simulink model "Electrical_System_2018b_obfs"  (R2019b)
settings: Solver=VariableStepAuto  StartTime=0.0  StopTime=5  RelTol=1e-3  AbsTol=1e-3  EnableMultiTasking=on
InitFcn:
  | Steady_State_Initialisation;
StopFcn:
  | %sscexplore(simlog);
  | %Logging
undefined symbols (not defined in the file): abrlhklxvp, aexgmhuedq, afmfmjnutg, afpphrjpnc, ahuxbyvruc, alarvljztt, amxnyqmnuw, aodrlwvqie, aolhmuplyq, aqpmguuqkg, auesgwirzl, aurophlnng, awamelrhru, ayfhvxflxn, azxkacuhqc, babszerikg, bawhdqanwq, bevoqecvei, bltjvqbchx, bmqsuewujl, bsmyqjfgnf, btvjbsmnve, bywgxqeadw, bziaduxaer, bzmcmdqocb, bzsvyvetat, ccsjnrbsih, cdvenygxwh, cedkrnslhx, cjheorclzs, cjrdshrtqx, ckhavyhcza, ckxewznhlz, cmrcgyiplk, conenicnws, cqkejbgjnn, csfnuwymhe, cunupkhwbh, cwzfvzuxxh, dcadmadufn, dcfponivnv, ddtrqjrhjn, dfhoxvkqas, dfrhtcwpne, dfvomcagjv, djijwylxea, dnmeqksrrm, dnzewbdkaa, dsqcykyxav, dtswwlttmm, ecumpidjtv, edegaywrct, ejjjsmnejc, eknqnehjdz, emvdetzouf, esxbqkbahr, etnkkbreiq, eunoiiiirw, ewewcuedir, fatkfxdhtc ... (+386)
libraries: fl_lib x802, ee_lib x362, fl_ps_legacy_lib x160, nesl_utility x85
(part 3 of 26)

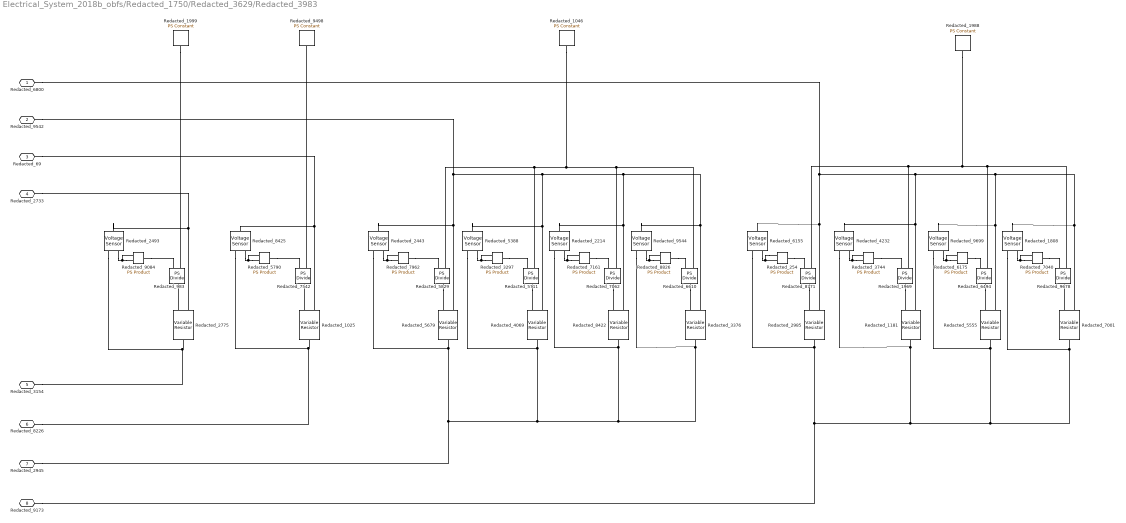
== system Electrical_System_2018b_obfs/Redacted_1750/Redacted_3629/Redacted_3983 ==
  Redacted_1025 : fl_lib/Electrical/Electrical Elements/Variable Resistor  Rmin=qncggggexc Ohm  i_specify=off  i_priority=None  i=gwvltjgfle A  i_nominal_specify=off  i_nominal_unit=A  i_nominal_value=ddwygaqqls  v_specify=off  v_priority=None  v=xwdlpdmsta V  v_nominal_specify=off  v_nominal_unit=V  v_nominal_value=czztgpkpzk
  Redacted_1046 : fl_lib/Physical Signals/Sources/PS Constant  constant=yrrhxgjxjc
  Redacted_1181 : fl_lib/Electrical/Electrical Elements/Variable Resistor  Rmin=nictvldxmh Ohm  i_specify=off  i_priority=None  i=znkaguzczs A  i_nominal_specify=off  i_nominal_unit=A  i_nominal_value=gwvbwqzrqi  v_specify=off  v_priority=None  v=zswwklaalm V  v_nominal_specify=off  v_nominal_unit=V  v_nominal_value=yhsekcleki
  Redacted_{1808,2214,2443,2493,4232,5388,6155,8425,9544,9699} (10 alike) : fl_lib/Electrical/Electrical Sensors/Voltage Sensor
  Redacted_{983,1969,5711,5829,6494,6610,7062,7542,8771,9678} (10 alike) : fl_ps_legacy_lib/Legacy Physical Signals/Functions/PS Divide
      settings: SourceProductName=Simscape  SourceProductBaseCode=SS  InternalSimscapePortConfiguration="{\"Bottom\":[],\"Left\":[{\"id\":\"I1\",\"label\":\"\",\"type\":\"input\"},{\"id\":\"I2\",\"label\":\"\",\"type\":\"input\"}],\"Right\":[{\"id\":\"O\",\"label\":\"\",\"type\":\"output\"}],\"Top\":[]}"
  Redacted_1988 : fl_lib/Physical Signals/Sources/PS Constant  constant=dwzkorkybi
  Redacted_1999 : fl_lib/Physical Signals/Sources/PS Constant  constant=qaltaheucg
  Redacted_{254,3297,3744,5790,6175,7040,7161,7962,8826,9084} (10 alike) : fl_ps_legacy_lib/Legacy Physical Signals/Functions/PS Product
      settings: SourceProductName=Simscape  SourceProductBaseCode=SS
  Redacted_2775 : fl_lib/Electrical/Electrical Elements/Variable Resistor  Rmin=reyjghhurh Ohm  i_specify=off  i_priority=None  i=fnfcgkgufq A  i_nominal_specify=off  i_nominal_unit=A  i_nominal_value=ruiumlemge  v_specify=off  v_priority=None  v=rpfslwjagr V  v_nominal_specify=off  v_nominal_unit=V  v_nominal_value=kprgkhsdzv
  Redacted_2985 : fl_lib/Electrical/Electrical Elements/Variable Resistor  Rmin=opektvarcr Ohm  i_specify=off  i_priority=None  i=ipmwytsvba A  i_nominal_specify=off  i_nominal_unit=A  i_nominal_value=zmaalwbitl  v_specify=off  v_priority=None  v=mourxlmgxq V  v_nominal_specify=off  v_nominal_unit=V  v_nominal_value=olwmmtumto
  Redacted_3376 : fl_lib/Electrical/Electrical Elements/Variable Resistor  Rmin=dmoucclhwu Ohm  i_specify=off  i_priority=None  i=qsvqtyyrfy A  i_nominal_specify=off  i_nominal_unit=A  i_nominal_value=ejaoihdkoa  v_specify=off  v_priority=None  v=bjbzrdorum V  v_nominal_specify=off  v_nominal_unit=V  v_nominal_value=hihsrnonml
  Redacted_4069 : fl_lib/Electrical/Electrical Elements/Variable Resistor  Rmin=bbvrroiejc Ohm  i_specify=off  i_priority=None  i=wnccttposb A  i_nominal_specify=off  i_nominal_unit=A  i_nominal_value=dxfjwicvev  v_specify=off  v_priority=None  v=rbnooizcor V  v_nominal_specify=off  v_nominal_unit=V  v_nominal_value=vmgjehqswm
  Redacted_5555 : fl_lib/Electrical/Electrical Elements/Variable Resistor  Rmin=dsgwiuwtzd Ohm  i_specify=off  i_priority=None  i=qbydpwndjg A  i_nominal_specify=off  i_nominal_unit=A  i_nominal_value=olcbtcjicg  v_specify=off  v_priority=None  v=jvfxdepjcq V  v_nominal_specify=off  v_nominal_unit=V  v_nominal_value=claoggoaet
  Redacted_5679 : fl_lib/Electrical/Electrical Elements/Variable Resistor  Rmin=alpgflrfvh Ohm  i_specify=off  i_priority=None  i=hhwawqdbpi A  i_nominal_specify=off  i_nominal_unit=A  i_nominal_value=hmlbwyynal  v_specify=off  v_priority=None  v=mblpeolwgc V  v_nominal_specify=off  v_nominal_unit=V  v_nominal_value=fswqhenwkq
  Redacted_7001 : fl_lib/Electrical/Electrical Elements/Variable Resistor  Rmin=wojwfybect Ohm  i_specify=off  i_priority=None  i=cubmhvxrnv A  i_nominal_specify=off  i_nominal_unit=A  i_nominal_value=jjakzqrkrp  v_specify=off  v_priority=None  v=kgoihxmpfv V  v_nominal_specify=off  v_nominal_unit=V  v_nominal_value=dzhpomehap
  Redacted_8422 : fl_lib/Electrical/Electrical Elements/Variable Resistor  Rmin=eatydowpoa Ohm  i_specify=off  i_priority=None  i=pfhnarewmr A  i_nominal_specify=off  i_nominal_unit=A  i_nominal_value=mvkwcnovui  v_specify=off  v_priority=None  v=vbpjazytgn V  v_nominal_specify=off  v_nominal_unit=V  v_nominal_value=ttjtmxbkxy
  Redacted_9498 : fl_lib/Physical Signals/Sources/PS Constant  constant=ljceyavbcj
  Redacted_6800 : PMIOPort  Side=Left
  Redacted_9542 : PMIOPort  Port=2  Side=Left
  Redacted_69 : PMIOPort  Port=3  Side=Left
  Redacted_2733 : PMIOPort  Port=4  Side=Left
  Redacted_3154 : PMIOPort  Port=5  Side=Left
  Redacted_8226 : PMIOPort  Port=6  Side=Left
  Redacted_2945 : PMIOPort  Port=7  Side=Left
  Redacted_9173 : PMIOPort  Port=8  Side=Left
  connections:
  Redacted_254/LConn1 -- Redacted_254/LConn2 -- Redacted_6155/RConn1
  Redacted_3744/LConn2 -- Redacted_3744/LConn1 -- Redacted_4232/RConn1
  Redacted_6494/LConn2 -- Redacted_9678/LConn2 -- Redacted_1988/RConn1 -- Redacted_8771/LConn2 -- Redacted_1969/LConn2
  Redacted_5679/RConn1 -- Redacted_2443/RConn2 -- Redacted_2945/RConn1 -- Redacted_9544/RConn2 -- Redacted_3376/RConn1 -- Redacted_2214/RConn2 -- Redacted_8422/RConn1 -- Redacted_4069/RConn1 -- Redacted_5388/RConn2
  Redacted_1025/LConn2 -- Redacted_8425/LConn1 -- Redacted_69/RConn1
  Redacted_1181/LConn2 -- Redacted_4232/LConn1 -- Redacted_6800/RConn1 -- Redacted_6155/LConn1 -- Redacted_2985/LConn2 -- Redacted_1808/LConn1 -- Redacted_7001/LConn2 -- Redacted_5555/LConn2 -- Redacted_9699/LConn1
  Redacted_2493/RConn2 -- Redacted_2775/RConn1 -- Redacted_3154/RConn1
  Redacted_8425/RConn2 -- Redacted_1025/RConn1 -- Redacted_8226/RConn1
  Redacted_8826/LConn2 -- Redacted_8826/LConn1 -- Redacted_9544/RConn1
  Redacted_9699/RConn2 -- Redacted_5555/RConn1 -- Redacted_9173/RConn1 -- Redacted_2985/RConn1 -- Redacted_6155/RConn2 -- Redacted_4232/RConn2 -- Redacted_1181/RConn1 -- Redacted_7001/RConn1 -- Redacted_1808/RConn2
  Redacted_5790/LConn2 -- Redacted_5790/LConn1 -- Redacted_8425/RConn1
  Redacted_7040/LConn2 -- Redacted_7040/LConn1 -- Redacted_1808/RConn1
  Redacted_2214/LConn1 -- Redacted_8422/LConn2 -- Redacted_9544/LConn1 -- Redacted_3376/LConn2 -- Redacted_4069/LConn2 -- Redacted_5388/LConn1 -- Redacted_9542/RConn1 -- Redacted_5679/LConn2 -- Redacted_2443/LConn1
  Redacted_3297/LConn2 -- Redacted_3297/LConn1 -- Redacted_5388/RConn1
  Redacted_7062/LConn2 -- Redacted_6610/LConn2 -- Redacted_1046/RConn1 -- Redacted_5829/LConn2 -- Redacted_5711/LConn2
  Redacted_2493/LConn1 -- Redacted_2775/LConn2 -- Redacted_2733/RConn1
  Redacted_7161/LConn2 -- Redacted_7161/LConn1 -- Redacted_2214/RConn1
  Redacted_9084/LConn2 -- Redacted_9084/LConn1 -- Redacted_2493/RConn1
  Redacted_7962/LConn2 -- Redacted_7962/LConn1 -- Redacted_2443/RConn1
  Redacted_6175/LConn2 -- Redacted_6175/LConn1 -- Redacted_9699/RConn1
  Redacted_3297/RConn1 -- Redacted_5711/LConn1
  Redacted_1025/LConn1 -- Redacted_7542/RConn1
  Redacted_3744/RConn1 -- Redacted_1969/LConn1
  Redacted_6175/RConn1 -- Redacted_6494/LConn1
  Redacted_5829/RConn1 -- Redacted_5679/LConn1
  Redacted_1969/RConn1 -- Redacted_1181/LConn1
  Redacted_9084/RConn1 -- Redacted_983/LConn1
  Redacted_7161/RConn1 -- Redacted_7062/LConn1
  Redacted_8771/RConn1 -- Redacted_2985/LConn1
  Redacted_8826/RConn1 -- Redacted_6610/LConn1
  Redacted_7542/LConn2 -- Redacted_9498/RConn1
  Redacted_254/RConn1 -- Redacted_8771/LConn1
  Redacted_2775/LConn1 -- Redacted_983/RConn1
  Redacted_1999/RConn1 -- Redacted_983/LConn2
  Redacted_7001/LConn1 -- Redacted_9678/RConn1
  Redacted_5711/RConn1 -- Redacted_4069/LConn1
  Redacted_7962/RConn1 -- Redacted_5829/LConn1
  Redacted_6494/RConn1 -- Redacted_5555/LConn1
  Redacted_7062/RConn1 -- Redacted_8422/LConn1
  Redacted_5790/RConn1 -- Redacted_7542/LConn1
  Redacted_6610/RConn1 -- Redacted_3376/LConn1
  Redacted_7040/RConn1 -- Redacted_9678/LConn1

== system Electrical_System_2018b_obfs/Redacted_1750/Redacted_393/Redacted_3640 ==
  Redacted_1716 : fl_lib/Physical Signals/Sources/PS Constant  constant=mmajduezkq
  Redacted_199 : fl_ps_legacy_lib/Legacy Physical Signals/Functions/PS Divide
      settings: SourceProductName=Simscape  SourceProductBaseCode=SS  InternalSimscapePortConfiguration="{\"Bottom\":[],\"Left\":[{\"id\":\"I1\",\"label\":\"\",\"type\":\"input\"},{\"id\":\"I2\",\"label\":\"\",\"type\":\"input\"}],\"Right\":[{\"id\":\"O\",\"label\":\"\",\"type\":\"output\"}],\"Top\":[]}"
  Redacted_4562 : fl_lib/Electrical/Electrical Elements/Variable Resistor  Rmin=kdjcxtkztl Ohm  i_specify=off  i_priority=None  i=cqxgsgfmtn A  i_nominal_specify=off  i_nominal_unit=A  i_nominal_value=bklpitcnvv  v_specify=off  v_priority=None  v=hyuagysdcb V  v_nominal_specify=off  v_nominal_unit=V  v_nominal_value=etqsntubpw
  Redacted_4611 : fl_lib/Electrical/Electrical Elements/Variable Resistor  Rmin=tgyotuwxyj Ohm  i_specify=off  i_priority=None  i=ffbyfrgsin A  i_nominal_specify=off  i_nominal_unit=A  i_nominal_value=lmnpciehqe  v_specify=off  v_priority=None  v=veajvkhyvt V  v_nominal_specify=off  v_nominal_unit=V  v_nominal_value=boksjqkemi
  Redacted_4847 : fl_ps_legacy_lib/Legacy Physical Signals/Functions/PS Product
      settings: SourceProductName=Simscape  SourceProductBaseCode=SS
  Redacted_5241 : fl_lib/Physical Signals/Sources/PS Constant  constant=uldbrsmhhe
  Redacted_5245 : fl_lib/Electrical/Electrical Sensors/Voltage Sensor
  Redacted_6942 : fl_lib/Electrical/Electrical Sensors/Voltage Sensor
  Redacted_8381 : fl_ps_legacy_lib/Legacy Physical Signals/Functions/PS Divide
      settings: SourceProductName=Simscape  SourceProductBaseCode=SS  InternalSimscapePortConfiguration="{\"Bottom\":[],\"Left\":[{\"id\":\"I1\",\"label\":\"\",\"type\":\"input\"},{\"id\":\"I2\",\"label\":\"\",\"type\":\"input\"}],\"Right\":[{\"id\":\"O\",\"label\":\"\",\"type\":\"output\"}],\"Top\":[]}"
  Redacted_9241 : fl_ps_legacy_lib/Legacy Physical Signals/Functions/PS Product
      settings: SourceProductName=Simscape  SourceProductBaseCode=SS
  Redacted_8912 : PMIOPort  Side=Left
  Redacted_9942 : PMIOPort  Port=2  Side=Left
  Redacted_6824 : PMIOPort  Port=3  Side=Left
  Redacted_5238 : PMIOPort  Port=4  Side=Left
  connections:
  Redacted_9241/LConn1 -- Redacted_9241/LConn2 -- Redacted_6942/RConn1
  Redacted_6942/LConn1 -- Redacted_4562/LConn2 -- Redacted_8912/RConn1
  Redacted_5245/RConn2 -- Redacted_4611/RConn1 -- Redacted_6824/RConn1
  Redacted_4847/LConn1 -- Redacted_5245/RConn1 -- Redacted_4847/LConn2
  Redacted_4562/RConn1 -- Redacted_6942/RConn2 -- Redacted_5238/RConn1
  Redacted_5245/LConn1 -- Redacted_4611/LConn2 -- Redacted_9942/RConn1
  Redacted_8381/LConn2 -- Redacted_5241/RConn1
  Redacted_199/RConn1 -- Redacted_4562/LConn1
  Redacted_9241/RConn1 -- Redacted_199/LConn1
  Redacted_4847/RConn1 -- Redacted_8381/LConn1
  Redacted_1716/RConn1 -- Redacted_199/LConn2
  Redacted_8381/RConn1 -- Redacted_4611/LConn1

== system Electrical_System_2018b_obfs/Redacted_1750/Redacted_418/Redacted_6987 ==
  Redacted_2047 : fl_lib/Electrical/Electrical Elements/Variable Resistor  Rmin=lauxoojxid Ohm  i_specify=off  i_priority=None  i=plucywvrmo A  i_nominal_specify=off  i_nominal_unit=A  i_nominal_value=pntbnmmjvt  v_specify=off  v_priority=None  v=exyxduxjmg V  v_nominal_specify=off  v_nominal_unit=V  v_nominal_value=uxkjompdua
  Redacted_2337 : fl_lib/Electrical/Electrical Sensors/Voltage Sensor
  Redacted_2505 : fl_lib/Electrical/Electrical Elements/Variable Resistor  Rmin=vmtqcufeiw Ohm  i_specify=off  i_priority=None  i=jdptkrmseg A  i_nominal_specify=off  i_nominal_unit=A  i_nominal_value=gpzxlmwhqh  v_specify=off  v_priority=None  v=yfdhwgbouy V  v_nominal_specify=off  v_nominal_unit=V  v_nominal_value=fbrxqazbqz
  Redacted_2649 : fl_lib/Physical Signals/Sources/PS Constant  constant=oimdssqwfz
  Redacted_3101 : fl_ps_legacy_lib/Legacy Physical Signals/Functions/PS Divide
      settings: SourceProductName=Simscape  SourceProductBaseCode=SS  InternalSimscapePortConfiguration="{\"Bottom\":[],\"Left\":[{\"id\":\"I1\",\"label\":\"\",\"type\":\"input\"},{\"id\":\"I2\",\"label\":\"\",\"type\":\"input\"}],\"Right\":[{\"id\":\"O\",\"label\":\"\",\"type\":\"output\"}],\"Top\":[]}"
  Redacted_4326 : fl_ps_legacy_lib/Legacy Physical Signals/Functions/PS Product
      settings: SourceProductName=Simscape  SourceProductBaseCode=SS
  Redacted_6351 : fl_lib/Physical Signals/Sources/PS Constant  constant=bognseoxqa
  Redacted_7217 : fl_ps_legacy_lib/Legacy Physical Signals/Functions/PS Divide
      settings: SourceProductName=Simscape  SourceProductBaseCode=SS  InternalSimscapePortConfiguration="{\"Bottom\":[],\"Left\":[{\"id\":\"I1\",\"label\":\"\",\"type\":\"input\"},{\"id\":\"I2\",\"label\":\"\",\"type\":\"input\"}],\"Right\":[{\"id\":\"O\",\"label\":\"\",\"type\":\"output\"}],\"Top\":[]}"
  Redacted_7328 : fl_lib/Electrical/Electrical Sensors/Voltage Sensor
  Redacted_9391 : fl_ps_legacy_lib/Legacy Physical Signals/Functions/PS Product
      settings: SourceProductName=Simscape  SourceProductBaseCode=SS
  Redacted_1593 : PMIOPort  Side=Left
  Redacted_8573 : PMIOPort  Port=2  Side=Left
  Redacted_2123 : PMIOPort  Port=3  Side=Left
  Redacted_5119 : PMIOPort  Port=4  Side=Left
  connections:
  Redacted_9391/LConn1 -- Redacted_9391/LConn2 -- Redacted_2337/RConn1
  Redacted_2337/LConn1 -- Redacted_2047/LConn2 -- Redacted_1593/RConn1
  Redacted_7328/RConn2 -- Redacted_2505/RConn1 -- Redacted_2123/RConn1
  Redacted_4326/LConn1 -- Redacted_7328/RConn1 -- Redacted_4326/LConn2
  Redacted_2047/RConn1 -- Redacted_2337/RConn2 -- Redacted_5119/RConn1
  Redacted_7328/LConn1 -- Redacted_2505/LConn2 -- Redacted_8573/RConn1
  Redacted_7217/LConn2 -- Redacted_2649/RConn1
  Redacted_3101/RConn1 -- Redacted_2047/LConn1
  Redacted_9391/RConn1 -- Redacted_3101/LConn1
  Redacted_4326/RConn1 -- Redacted_7217/LConn1
  Redacted_6351/RConn1 -- Redacted_3101/LConn2
  Redacted_7217/RConn1 -- Redacted_2505/LConn1

== system Electrical_System_2018b_obfs/Redacted_1750/Redacted_5682/Redacted_8066 ==
  Redacted_1177 : fl_lib/Electrical/Electrical Elements/Variable Resistor  Rmin=vkyvigtamz Ohm  i_specify=off  i_priority=None  i=wppjqmzgdt A  i_nominal_specify=off  i_nominal_unit=A  i_nominal_value=lkbsnljfkr  v_specify=off  v_priority=None  v=qpdznmgncc V  v_nominal_specify=off  v_nominal_unit=V  v_nominal_value=vudvbbkcaq
  Redacted_{142,2192,4682,9058} (4 alike) : fl_lib/Electrical/Electrical Sensors/Voltage Sensor
  Redacted_1746 : fl_lib/Physical Signals/Sources/PS Constant  constant=qszgelsouu
  Redacted_1854 : fl_lib/Electrical/Electrical Elements/Variable Resistor  Rmin=kiuysncemq Ohm  i_specify=off  i_priority=None  i=lroptwomwf A  i_nominal_specify=off  i_nominal_unit=A  i_nominal_value=trlhttlhbq  v_specify=off  v_priority=None  v=rbkqrozlms V  v_nominal_specify=off  v_nominal_unit=V  v_nominal_value=dnncgyeoix
  Redacted_{2912,7599,8120,9137} (4 alike) : fl_ps_legacy_lib/Legacy Physical Signals/Functions/PS Divide
      settings: SourceProductName=Simscape  SourceProductBaseCode=SS  InternalSimscapePortConfiguration="{\"Bottom\":[],\"Left\":[{\"id\":\"I1\",\"label\":\"\",\"type\":\"input\"},{\"id\":\"I2\",\"label\":\"\",\"type\":\"input\"}],\"Right\":[{\"id\":\"O\",\"label\":\"\",\"type\":\"output\"}],\"Top\":[]}"
  Redacted_309 : fl_lib/Electrical/Electrical Elements/Variable Resistor  Rmin=hxkyfdhnhj Ohm  i_specify=off  i_priority=None  i=hnfietiele A  i_nominal_specify=off  i_nominal_unit=A  i_nominal_value=mykgswtkce  v_specify=off  v_priority=None  v=kwhtknwfyy V  v_nominal_specify=off  v_nominal_unit=V  v_nominal_value=vkmosjkefd
  Redacted_324 : fl_lib/Electrical/Electrical Elements/Variable Resistor  Rmin=gxqnvagobp Ohm  i_specify=off  i_priority=None  i=qrtnkfnhvu A  i_nominal_specify=off  i_nominal_unit=A  i_nominal_value=kknzxrhjtc  v_specify=off  v_priority=None  v=isvapyiliw V  v_nominal_specify=off  v_nominal_unit=V  v_nominal_value=xsrfklrfwh
  Redacted_{3820,4656,5258,5308} (4 alike) : fl_ps_legacy_lib/Legacy Physical Signals/Functions/PS Product
      settings: SourceProductName=Simscape  SourceProductBaseCode=SS
  Redacted_4042 : fl_lib/Physical Signals/Sources/PS Constant  constant=kzfpfybhsi
  Redacted_4697 : fl_lib/Physical Signals/Sources/PS Constant  constant=hmemlihtnk
  Redacted_8018 : fl_lib/Physical Signals/Sources/PS Constant  constant=yfikxvaohm
  Redacted_9895 : PMIOPort  Side=Left
  Redacted_6360 : PMIOPort  Port=2  Side=Left
  Redacted_7645 : PMIOPort  Port=3  Side=Left
  Redacted_2461 : PMIOPort  Port=4  Side=Left
  Redacted_3445 : PMIOPort  Port=5  Side=Right
  Redacted_5329 : PMIOPort  Port=6  Side=Right
  Redacted_8781 : PMIOPort  Port=7  Side=Right
  Redacted_5062 : PMIOPort  Port=8  Side=Right
  connections:
  Redacted_142/RConn1 -- Redacted_5308/LConn2 -- Redacted_5308/LConn1
  Redacted_3820/LConn2 -- Redacted_2192/RConn1 -- Redacted_3820/LConn1
  Redacted_9058/RConn1 -- Redacted_4656/LConn2 -- Redacted_4656/LConn1
  Redacted_5258/LConn2 -- Redacted_4682/RConn1 -- Redacted_5258/LConn1
  Redacted_142/RConn2 -- Redacted_1177/RConn1 -- Redacted_7645/RConn1
  Redacted_142/LConn1 -- Redacted_1177/LConn2 -- Redacted_6360/RConn1
  Redacted_2192/LConn1 -- Redacted_324/LConn2 -- Redacted_5329/RConn1
  Redacted_4682/LConn1 -- Redacted_1854/LConn2 -- Redacted_9895/RConn1
  Redacted_309/RConn1 -- Redacted_9058/RConn2 -- Redacted_5062/RConn1
  Redacted_9058/LConn1 -- Redacted_309/LConn2 -- Redacted_3445/RConn1
  Redacted_4682/RConn2 -- Redacted_1854/RConn1 -- Redacted_2461/RConn1
  Redacted_324/RConn1 -- Redacted_2192/RConn2 -- Redacted_8781/RConn1
  Redacted_8120/LConn2 -- Redacted_4042/RConn1
  Redacted_7599/LConn2 -- Redacted_1746/RConn1
  Redacted_5258/RConn1 -- Redacted_7599/LConn1
  Redacted_9137/LConn2 -- Redacted_4697/RConn1
  Redacted_324/LConn1 -- Redacted_2912/RConn1
  Redacted_4656/RConn1 -- Redacted_8120/LConn1
  Redacted_2912/LConn2 -- Redacted_8018/RConn1
  Redacted_309/LConn1 -- Redacted_8120/RConn1
  Redacted_5308/RConn1 -- Redacted_9137/LConn1
  Redacted_1177/LConn1 -- Redacted_9137/RConn1
  Redacted_1854/LConn1 -- Redacted_7599/RConn1
  Redacted_3820/RConn1 -- Redacted_2912/LConn1

== system Electrical_System_2018b_obfs/Redacted_1750/Redacted_7456/Redacted_986 ==
  Redacted_3578 : fl_lib/Electrical/Electrical Sensors/Voltage Sensor
  Redacted_3630 : fl_lib/Physical Signals/Sources/PS Constant  constant=qbbmnonqyb
  Redacted_3749 : fl_ps_legacy_lib/Legacy Physical Signals/Functions/PS Product
      settings: SourceProductName=Simscape  SourceProductBaseCode=SS
  Redacted_4140 : fl_lib/Electrical/Electrical Elements/Variable Resistor  Rmin=vfyjjfyhxj Ohm  i_specify=off  i_priority=None  i=faygszjviu A  i_nominal_specify=off  i_nominal_unit=A  i_nominal_value=nqsiwtqwnm  v_specify=off  v_priority=None  v=hzkergozfv V  v_nominal_specify=off  v_nominal_unit=V  v_nominal_value=cpmedzmwhe
  Redacted_4316 : fl_ps_legacy_lib/Legacy Physical Signals/Functions/PS Divide
      settings: SourceProductName=Simscape  SourceProductBaseCode=SS  InternalSimscapePortConfiguration="{\"Bottom\":[],\"Left\":[{\"id\":\"I1\",\"label\":\"\",\"type\":\"input\"},{\"id\":\"I2\",\"label\":\"\",\"type\":\"input\"}],\"Right\":[{\"id\":\"O\",\"label\":\"\",\"type\":\"output\"}],\"Top\":[]}"
  Redacted_2977 : PMIOPort  Side=Left
  Redacted_8753 : PMIOPort  Port=2  Side=Left
  connections:
  Redacted_4140/RConn1 -- Redacted_8753/RConn1 -- Redacted_3578/RConn2
  Redacted_3578/RConn1 -- Redacted_3749/LConn2 -- Redacted_3749/LConn1
  Redacted_4140/LConn2 -- Redacted_2977/RConn1 -- Redacted_3578/LConn1
  Redacted_4316/LConn2 -- Redacted_3630/RConn1
  Redacted_3749/RConn1 -- Redacted_4316/LConn1
  Redacted_4316/RConn1 -- Redacted_4140/LConn1

== system Electrical_System_2018b_obfs/Redacted_1750/Redacted_7650/Redacted_6349 ==
  Redacted_{1234,1499,1809,1832,4046,4654,5172,5477,8721,9671} (10 alike) : fl_lib/Electrical/Electrical Sensors/Voltage Sensor
  Redacted_1255 : fl_lib/Electrical/Electrical Elements/Variable Resistor  Rmin=toajursngw Ohm  i_specify=off  i_priority=None  i=yfnidnbwwh A  i_nominal_specify=off  i_nominal_unit=A  i_nominal_value=zthunajpho  v_specify=off  v_priority=None  v=ifaghnzdys V  v_nominal_specify=off  v_nominal_unit=V  v_nominal_value=wixrfdgsuz
  Redacted_1446 : fl_lib/Electrical/Electrical Elements/Variable Resistor  Rmin=pzdknduoqo Ohm  i_specify=off  i_priority=None  i=oztilupibk A  i_nominal_specify=off  i_nominal_unit=A  i_nominal_value=rnqfwyptoq  v_specify=off  v_priority=None  v=ltuihodwwc V  v_nominal_specify=off  v_nominal_unit=V  v_nominal_value=ewsrtxtzen
  Redacted_{72,191,1466,2390,2485,3700,4694,8278,8363,9757} (10 alike) : fl_ps_legacy_lib/Legacy Physical Signals/Functions/PS Divide
      settings: SourceProductName=Simscape  SourceProductBaseCode=SS  InternalSimscapePortConfiguration="{\"Bottom\":[],\"Left\":[{\"id\":\"I1\",\"label\":\"\",\"type\":\"input\"},{\"id\":\"I2\",\"label\":\"\",\"type\":\"input\"}],\"Right\":[{\"id\":\"O\",\"label\":\"\",\"type\":\"output\"}],\"Top\":[]}"
  Redacted_1589 : fl_lib/Electrical/Electrical Elements/Variable Resistor  Rmin=izjqjwrvha Ohm  i_specify=off  i_priority=None  i=rphwujzcay A  i_nominal_specify=off  i_nominal_unit=A  i_nominal_value=zskshjause  v_specify=off  v_priority=None  v=vephavlban V  v_nominal_specify=off  v_nominal_unit=V  v_nominal_value=lpqimgyknq
  Redacted_{479,1734,2157,4074,6022,7316,7580,7985,9835,9939} (10 alike) : fl_ps_legacy_lib/Legacy Physical Signals/Functions/PS Product
      settings: SourceProductName=Simscape  SourceProductBaseCode=SS
  Redacted_2452 : fl_lib/Electrical/Electrical Elements/Variable Resistor  Rmin=aznchvcbsy Ohm  i_specify=off  i_priority=None  i=wcmnmikgyd A  i_nominal_specify=off  i_nominal_unit=A  i_nominal_value=cgeanztcbw  v_specify=off  v_priority=None  v=yxnsxguivt V  v_nominal_specify=off  v_nominal_unit=V  v_nominal_value=dhfptsawyg
  Redacted_2626 : fl_lib/Electrical/Electrical Elements/Variable Resistor  Rmin=jzssibrerx Ohm  i_specify=off  i_priority=None  i=ohsfembpji A  i_nominal_specify=off  i_nominal_unit=A  i_nominal_value=zdthborjez  v_specify=off  v_priority=None  v=uymwsamwyx V  v_nominal_specify=off  v_nominal_unit=V  v_nominal_value=pmsnpwidgf
  Redacted_3085 : fl_lib/Electrical/Electrical Elements/Variable Resistor  Rmin=xoqpzpdmhd Ohm  i_specify=off  i_priority=None  i=kxqlrdlpwd A  i_nominal_specify=off  i_nominal_unit=A  i_nominal_value=ywvqegruxx  v_specify=off  v_priority=None  v=ewcohjexxl V  v_nominal_specify=off  v_nominal_unit=V  v_nominal_value=mweodujhcn
  Redacted_3807 : fl_lib/Electrical/Electrical Elements/Variable Resistor  Rmin=japywzwbst Ohm  i_specify=off  i_priority=None  i=qmzonwdowz A  i_nominal_specify=off  i_nominal_unit=A  i_nominal_value=nouytsvqdq  v_specify=off  v_priority=None  v=tnfovutweq V  v_nominal_specify=off  v_nominal_unit=V  v_nominal_value=xcnuppncww
  Redacted_4269 : fl_lib/Electrical/Electrical Elements/Variable Resistor  Rmin=retlqzgpee Ohm  i_specify=off  i_priority=None  i=lbywahdzbx A  i_nominal_specify=off  i_nominal_unit=A  i_nominal_value=zdvgoejfjp  v_specify=off  v_priority=None  v=jrklsvsyak V  v_nominal_specify=off  v_nominal_unit=V  v_nominal_value=dxyztioorl
  Redacted_5256 : fl_lib/Physical Signals/Sources/PS Constant  constant=glgatpidjj
  Redacted_5721 : fl_lib/Electrical/Electrical Elements/Variable Resistor  Rmin=scjopjuxat Ohm  i_specify=off  i_priority=None  i=yjrzibxpwk A  i_nominal_specify=off  i_nominal_unit=A  i_nominal_value=ktpnmkyxfu  v_specify=off  v_priority=None  v=cqshxauyxy V  v_nominal_specify=off  v_nominal_unit=V  v_nominal_value=uzyxsspzoc
  Redacted_6728 : fl_lib/Physical Signals/Sources/PS Constant  constant=xdtdqlhagn
  Redacted_8070 : fl_lib/Physical Signals/Sources/PS Constant  constant=gocwlesmfg
  Redacted_8280 : fl_lib/Physical Signals/Sources/PS Constant  constant=auppxciawh
  Redacted_8701 : fl_lib/Electrical/Electrical Elements/Variable Resistor  Rmin=krsscguztg Ohm  i_specify=off  i_priority=None  i=qpjbswtkhu A  i_nominal_specify=off  i_nominal_unit=A  i_nominal_value=gmrnjlijvg  v_specify=off  v_priority=None  v=afdshqdvdz V  v_nominal_specify=off  v_nominal_unit=V  v_nominal_value=zfqdtjcjii
  Redacted_956 : PMIOPort  Side=Left
  Redacted_372 : PMIOPort  Port=2  Side=Left
  Redacted_7777 : PMIOPort  Port=3  Side=Left
  Redacted_2409 : PMIOPort  Port=4  Side=Left
  Redacted_4885 : PMIOPort  Port=5  Side=Left
  Redacted_8935 : PMIOPort  Port=6  Side=Left
  Redacted_4304 : PMIOPort  Port=7  Side=Left
  Redacted_3066 : PMIOPort  Port=8  Side=Left
  connections:
  Redacted_9939/LConn1 -- Redacted_9939/LConn2 -- Redacted_1832/RConn1
  Redacted_7316/LConn2 -- Redacted_7316/LConn1 -- Redacted_5172/RConn1
  Redacted_3700/LConn2 -- Redacted_1466/LConn2 -- Redacted_5256/RConn1 -- Redacted_2485/LConn2 -- Redacted_72/LConn2
  Redacted_2452/RConn1 -- Redacted_9671/RConn2 -- Redacted_4304/RConn1 -- Redacted_8721/RConn2 -- Redacted_1589/RConn1 -- Redacted_1499/RConn2 -- Redacted_5721/RConn1 -- Redacted_3807/RConn1 -- Redacted_1809/RConn2
  Redacted_4269/LConn2 -- Redacted_1234/LConn1 -- Redacted_7777/RConn1
  Redacted_1446/LConn2 -- Redacted_5172/LConn1 -- Redacted_956/RConn1 -- Redacted_1832/LConn1 -- Redacted_3085/LConn2 -- Redacted_4654/LConn1 -- Redacted_1255/LConn2 -- Redacted_2626/LConn2 -- Redacted_4046/LConn1
  Redacted_5477/RConn2 -- Redacted_8701/RConn1 -- Redacted_4885/RConn1
  Redacted_1234/RConn2 -- Redacted_4269/RConn1 -- Redacted_8935/RConn1
  Redacted_7985/LConn2 -- Redacted_7985/LConn1 -- Redacted_8721/RConn1
  Redacted_4046/RConn2 -- Redacted_2626/RConn1 -- Redacted_3066/RConn1 -- Redacted_3085/RConn1 -- Redacted_1832/RConn2 -- Redacted_5172/RConn2 -- Redacted_1446/RConn1 -- Redacted_1255/RConn1 -- Redacted_4654/RConn2
  Redacted_2157/LConn2 -- Redacted_2157/LConn1 -- Redacted_1234/RConn1
  Redacted_7580/LConn2 -- Redacted_7580/LConn1 -- Redacted_4654/RConn1
  Redacted_1499/LConn1 -- Redacted_5721/LConn2 -- Redacted_8721/LConn1 -- Redacted_1589/LConn2 -- Redacted_3807/LConn2 -- Redacted_1809/LConn1 -- Redacted_372/RConn1 -- Redacted_2452/LConn2 -- Redacted_9671/LConn1
  Redacted_1734/LConn2 -- Redacted_1734/LConn1 -- Redacted_1809/RConn1
  Redacted_8363/LConn2 -- Redacted_8278/LConn2 -- Redacted_8280/RConn1 -- Redacted_9757/LConn2 -- Redacted_2390/LConn2
  Redacted_5477/LConn1 -- Redacted_8701/LConn2 -- Redacted_2409/RConn1
  Redacted_9835/LConn2 -- Redacted_9835/LConn1 -- Redacted_1499/RConn1
  Redacted_4074/LConn2 -- Redacted_4074/LConn1 -- Redacted_5477/RConn1
  Redacted_479/LConn2 -- Redacted_479/LConn1 -- Redacted_9671/RConn1
  Redacted_6022/LConn2 -- Redacted_6022/LConn1 -- Redacted_4046/RConn1
  Redacted_1734/RConn1 -- Redacted_2390/LConn1
  Redacted_4269/LConn1 -- Redacted_191/RConn1
  Redacted_7316/RConn1 -- Redacted_72/LConn1
  Redacted_6022/RConn1 -- Redacted_3700/LConn1
  Redacted_9757/RConn1 -- Redacted_2452/LConn1
  Redacted_72/RConn1 -- Redacted_1446/LConn1
  Redacted_4074/RConn1 -- Redacted_4694/LConn1
  Redacted_9835/RConn1 -- Redacted_8363/LConn1
  Redacted_2485/RConn1 -- Redacted_3085/LConn1
  Redacted_7985/RConn1 -- Redacted_8278/LConn1
  Redacted_191/LConn2 -- Redacted_6728/RConn1
  Redacted_9939/RConn1 -- Redacted_2485/LConn1
  Redacted_8701/LConn1 -- Redacted_4694/RConn1
  Redacted_8070/RConn1 -- Redacted_4694/LConn2
  Redacted_1255/LConn1 -- Redacted_1466/RConn1
  Redacted_2390/RConn1 -- Redacted_3807/LConn1
  Redacted_479/RConn1 -- Redacted_9757/LConn1
  Redacted_3700/RConn1 -- Redacted_2626/LConn1
  Redacted_8363/RConn1 -- Redacted_5721/LConn1
  Redacted_2157/RConn1 -- Redacted_191/LConn1
  Redacted_8278/RConn1 -- Redacted_1589/LConn1
  Redacted_7580/RConn1 -- Redacted_1466/LConn1

== system Electrical_System_2018b_obfs/Redacted_1750/Redacted_8299/Redacted_4710 ==
  Redacted_137 : fl_lib/Electrical/Electrical Sensors/Voltage Sensor
  Redacted_1604 : fl_lib/Physical Signals/Sources/PS Constant  constant=bbfcyptcuo
  Redacted_167 : fl_lib/Electrical/Electrical Sensors/Voltage Sensor
  Redacted_2227 : fl_lib/Electrical/Electrical Elements/Variable Resistor  Rmin=lztewobgts Ohm  i_specify=off  i_priority=None  i=vbuobucesj A  i_nominal_specify=off  i_nominal_unit=A  i_nominal_value=nhfrabnupu  v_specify=on  v_priority=None  v=qzjwhntsxq V  v_nominal_specify=off  v_nominal_unit=V  v_nominal_value=ruccpaedow
  Redacted_2862 : fl_ps_legacy_lib/Legacy Physical Signals/Functions/PS Product
      settings: SourceProductName=Simscape  SourceProductBaseCode=SS
  Redacted_3914 : fl_ps_legacy_lib/Legacy Physical Signals/Functions/PS Product
      settings: SourceProductName=Simscape  SourceProductBaseCode=SS
  Redacted_421 : fl_lib/Electrical/Electrical Elements/Variable Resistor  Rmin=htfmmiqztp Ohm  i_specify=off  i_priority=None  i=ivjlxeqypp A  i_nominal_specify=off  i_nominal_unit=A  i_nominal_value=fyapxmmijy  v_specify=on  v_priority=None  v=tgofwmqpim V  v_nominal_specify=off  v_nominal_unit=V  v_nominal_value=wcptjihisv
  Redacted_4634 : fl_lib/Electrical/Electrical Elements/Variable Resistor  Rmin=rimeumodjt Ohm  i_specify=off  i_priority=None  i=zbqoxhceyc A  i_nominal_specify=off  i_nominal_unit=A  i_nominal_value=pswmfqtxxz  v_specify=on  v_priority=None  v=xcknhzaziw V  v_nominal_specify=off  v_nominal_unit=V  v_nominal_value=nmimjvxdhv
  Redacted_4644 : fl_lib/Physical Signals/Sources/PS Constant  constant=hbyanflpwv
  Redacted_580 : fl_lib/Electrical/Electrical Sensors/Voltage Sensor
  Redacted_6073 : fl_ps_legacy_lib/Legacy Physical Signals/Functions/PS Divide
      settings: SourceProductName=Simscape  SourceProductBaseCode=SS  InternalSimscapePortConfiguration="{\"Bottom\":[],\"Left\":[{\"id\":\"I1\",\"label\":\"\",\"type\":\"input\"},{\"id\":\"I2\",\"label\":\"\",\"type\":\"input\"}],\"Right\":[{\"id\":\"O\",\"label\":\"\",\"type\":\"output\"}],\"Top\":[]}"
  Redacted_7550 : fl_ps_legacy_lib/Legacy Physical Signals/Functions/PS Divide
      settings: SourceProductName=Simscape  SourceProductBaseCode=SS  InternalSimscapePortConfiguration="{\"Bottom\":[],\"Left\":[{\"id\":\"I1\",\"label\":\"\",\"type\":\"input\"},{\"id\":\"I2\",\"label\":\"\",\"type\":\"input\"}],\"Right\":[{\"id\":\"O\",\"label\":\"\",\"type\":\"output\"}],\"Top\":[]}"
  Redacted_8913 : fl_ps_legacy_lib/Legacy Physical Signals/Functions/PS Product
      settings: SourceProductName=Simscape  SourceProductBaseCode=SS
  Redacted_9022 : fl_ps_legacy_lib/Legacy Physical Signals/Functions/PS Divide
      settings: SourceProductName=Simscape  SourceProductBaseCode=SS  InternalSimscapePortConfiguration="{\"Bottom\":[],\"Left\":[{\"id\":\"I1\",\"label\":\"\",\"type\":\"input\"},{\"id\":\"I2\",\"label\":\"\",\"type\":\"input\"}],\"Right\":[{\"id\":\"O\",\"label\":\"\",\"type\":\"output\"}],\"Top\":[]}"
  Redacted_9291 : fl_lib/Physical Signals/Sources/PS Constant  constant=vuiuunkakd
  Redacted_4573 : PMIOPort  Side=Left
  Redacted_1220 : PMIOPort  Port=2  Side=Left
  Redacted_2982 : PMIOPort  Port=3  Side=Left
  Redacted_3513 : PMIOPort  Port=4  Side=Left
  Redacted_6567 : PMIOPort  Port=5  Side=Left
  Redacted_5311 : PMIOPort  Port=6  Side=Left
  connections:
  Redacted_8913/LConn2 -- Redacted_137/RConn1 -- Redacted_8913/LConn1
  Redacted_4634/LConn2 -- Redacted_2982/RConn1 -- Redacted_137/LConn1
  Redacted_137/RConn2 -- Redacted_3513/RConn1 -- Redacted_4634/RConn1
  Redacted_5311/RConn1 -- Redacted_580/RConn2 -- Redacted_2227/RConn1
  Redacted_1220/RConn1 -- Redacted_167/LConn1 -- Redacted_421/LConn2
  Redacted_6567/RConn1 -- Redacted_421/RConn1 -- Redacted_167/RConn2
  Redacted_4573/RConn1 -- Redacted_2227/LConn2 -- Redacted_580/LConn1
  Redacted_3914/LConn1 -- Redacted_167/RConn1 -- Redacted_3914/LConn2
  Redacted_2862/LConn2 -- Redacted_580/RConn1 -- Redacted_2862/LConn1
  Redacted_9022/LConn2 -- Redacted_4644/RConn1
  Redacted_9022/RConn1 -- Redacted_4634/LConn1
  Redacted_8913/RConn1 -- Redacted_9022/LConn1
  Redacted_3914/RConn1 -- Redacted_7550/LConn1
  Redacted_9291/RConn1 -- Redacted_7550/LConn2
  Redacted_7550/RConn1 -- Redacted_421/LConn1
  Redacted_6073/RConn1 -- Redacted_2227/LConn1
  Redacted_2862/RConn1 -- Redacted_6073/LConn1
  Redacted_1604/RConn1 -- Redacted_6073/LConn2

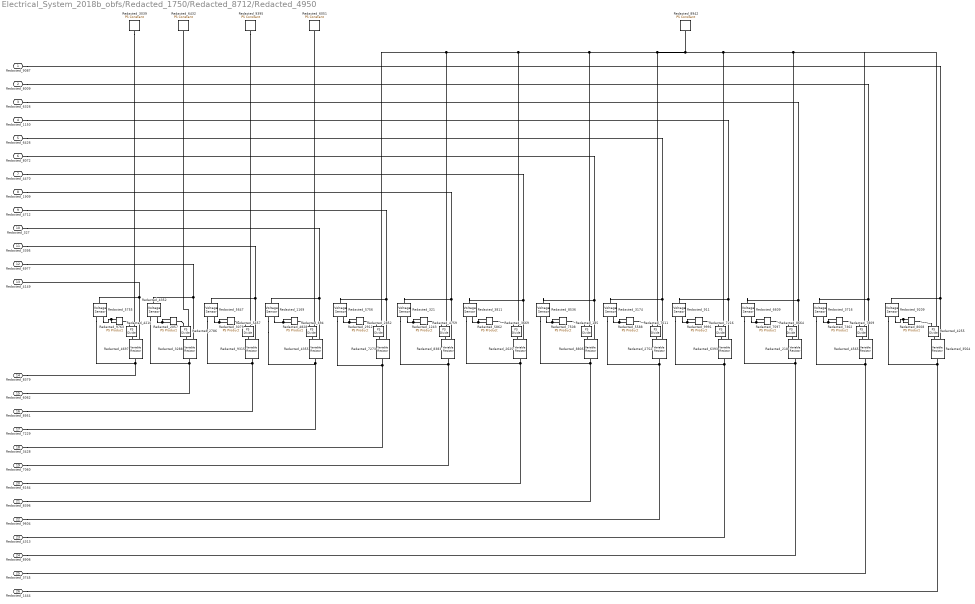
== system Electrical_System_2018b_obfs/Redacted_1750/Redacted_8712/Redacted_4950 ==
  Redacted_{321,911,1169,3174,3716,3811,4352,5647,5755..5756,6609,8536,9209} (13 alike) : fl_lib/Electrical/Electrical Sensors/Voltage Sensor
  Redacted_{1243,2057,2912,3079,4828,5588,5862,7362,7508,7597,8008,9763,9991} (13 alike) : fl_ps_legacy_lib/Legacy Physical Signals/Functions/PS Product
      settings: SourceProductName=Simscape  SourceProductBaseCode=SS
  Redacted_{185,694,2786,2852,3669,4210,4255,4759,5457,7011,7216,7809,8664} (13 alike) : fl_ps_legacy_lib/Legacy Physical Signals/Functions/PS Divide
      settings: SourceProductName=Simscape  SourceProductBaseCode=SS  InternalSimscapePortConfiguration="{\"Bottom\":[],\"Left\":[{\"id\":\"I1\",\"label\":\"\",\"type\":\"input\"},{\"id\":\"I2\",\"label\":\"\",\"type\":\"input\"}],\"Right\":[{\"id\":\"O\",\"label\":\"\",\"type\":\"output\"}],\"Top\":[]}"
  Redacted_218 : fl_lib/Electrical/Electrical Elements/Variable Resistor  Rmin=xkpevdmcbz Ohm  i_specify=off  i_priority=None  i=uqsrgcsonq A  i_nominal_specify=off  i_nominal_unit=A  i_nominal_value=lkzsewwykk  v_specify=off  v_priority=None  v=yotnplrabn V  v_nominal_specify=off  v_nominal_unit=V  v_nominal_value=woioxtpizx
  Redacted_2625 : fl_lib/Electrical/Electrical Elements/Variable Resistor  Rmin=iamqkpfczj Ohm  i_specify=off  i_priority=None  i=gruiwsozkt A  i_nominal_specify=off  i_nominal_unit=A  i_nominal_value=zgtzgsiamk  v_specify=off  v_priority=None  v=uvkvnqdmhx V  v_nominal_specify=off  v_nominal_unit=V  v_nominal_value=acjnbwmkge
  Redacted_2752 : fl_lib/Electrical/Electrical Elements/Variable Resistor  Rmin=rqfhnlzvvh Ohm  i_specify=off  i_priority=None  i=rsdrzjdeul A  i_nominal_specify=off  i_nominal_unit=A  i_nominal_value=jbtgkiqnwn  v_specify=off  v_priority=None  v=gydgulodds V  v_nominal_specify=off  v_nominal_unit=V  v_nominal_value=kpsofhlzmi
  Redacted_3039 : fl_lib/Physical Signals/Sources/PS Constant  constant=hayslkjznr
  Redacted_3288 : fl_lib/Electrical/Electrical Elements/Variable Resistor  Rmin=bfepvkbzxt Ohm  i_specify=off  i_priority=None  i=bixrkitofq A  i_nominal_specify=off  i_nominal_unit=A  i_nominal_value=pzvfxqeptj  v_specify=off  v_priority=None  v=hrfgfkfsgm V  v_nominal_specify=off  v_nominal_unit=V  v_nominal_value=abfxblzuku
  Redacted_3564 : fl_lib/Electrical/Electrical Elements/Variable Resistor  Rmin=swuyinsoxb Ohm  i_specify=off  i_priority=None  i=rtspcaxhwd A  i_nominal_specify=off  i_nominal_unit=A  i_nominal_value=endnrfokyx  v_specify=off  v_priority=None  v=ieeuzgftjx V  v_nominal_specify=off  v_nominal_unit=V  v_nominal_value=rzbuthgwfz
  Redacted_4355 : fl_lib/Electrical/Electrical Elements/Variable Resistor  Rmin=wjqooknifz Ohm  i_specify=off  i_priority=None  i=gtoodrgjqq A  i_nominal_specify=off  i_nominal_unit=A  i_nominal_value=sywuupkxsw  v_specify=off  v_priority=None  v=nczvbaurds V  v_nominal_specify=off  v_nominal_unit=V  v_nominal_value=vzeyifcwfq
  Redacted_4565 : fl_lib/Electrical/Electrical Elements/Variable Resistor  Rmin=mudoykpqdd Ohm  i_specify=off  i_priority=None  i=uflnxiwwiy A  i_nominal_specify=off  i_nominal_unit=A  i_nominal_value=uiqgnshhuz  v_specify=off  v_priority=None  v=yfwjpqdavk V  v_nominal_specify=off  v_nominal_unit=V  v_nominal_value=mpfpaxbmth
  Redacted_4697 : fl_lib/Electrical/Electrical Elements/Variable Resistor  Rmin=surzoqrfau Ohm  i_specify=off  i_priority=None  i=cqtvuzfoqx A  i_nominal_specify=off  i_nominal_unit=A  i_nominal_value=grwsvhkqec  v_specify=off  v_priority=None  v=rpvswoiusq V  v_nominal_specify=off  v_nominal_unit=V  v_nominal_value=wetkdncexg
  Redacted_6051 : fl_lib/Physical Signals/Sources/PS Constant  constant=yewurytqgn
  Redacted_6393 : fl_lib/Electrical/Electrical Elements/Variable Resistor  Rmin=chukkxztdl Ohm  i_specify=off  i_priority=None  i=ahklmzgqms A  i_nominal_specify=off  i_nominal_unit=A  i_nominal_value=kkoxaxegno  v_specify=off  v_priority=None  v=ajzeilyoqa V  v_nominal_specify=off  v_nominal_unit=V  v_nominal_value=gmlnjcxpku
  Redacted_6432 : fl_lib/Physical Signals/Sources/PS Constant  constant=emhqjlxzky
  Redacted_7273 : fl_lib/Electrical/Electrical Elements/Variable Resistor  Rmin=xdhkvwehbp Ohm  i_specify=off  i_priority=None  i=yzjazpcqtx A  i_nominal_specify=off  i_nominal_unit=A  i_nominal_value=ybqsbbhqdw  v_specify=off  v_priority=None  v=ewfqiywzdn V  v_nominal_specify=off  v_nominal_unit=V  v_nominal_value=jwpcggpkdg
  Redacted_8383 : fl_lib/Electrical/Electrical Elements/Variable Resistor  Rmin=hyagvbrnrb Ohm  i_specify=off  i_priority=None  i=eceuquddaw A  i_nominal_specify=off  i_nominal_unit=A  i_nominal_value=paczkwepjv  v_specify=off  v_priority=None  v=sbukybfgrr V  v_nominal_specify=off  v_nominal_unit=V  v_nominal_value=syqswvlqzq
  Redacted_8805 : fl_lib/Electrical/Electrical Elements/Variable Resistor  Rmin=pmsymaasaf Ohm  i_specify=off  i_priority=None  i=ynmaqmpxeu A  i_nominal_specify=off  i_nominal_unit=A  i_nominal_value=bczfbzwjff  v_specify=off  v_priority=None  v=iybikdqdai V  v_nominal_specify=off  v_nominal_unit=V  v_nominal_value=coqtebtvuk
  Redacted_8942 : fl_lib/Physical Signals/Sources/PS Constant  constant=gjekiqmrmz
  Redacted_9315 : fl_lib/Electrical/Electrical Elements/Variable Resistor  Rmin=heexyndvii Ohm  i_specify=off  i_priority=None  i=pkeqasscsd A  i_nominal_specify=off  i_nominal_unit=A  i_nominal_value=fuxkzhslqw  v_specify=off  v_priority=None  v=zjmqnwnmyg V  v_nominal_specify=off  v_nominal_unit=V  v_nominal_value=phbscrjmyh
  Redacted_9395 : fl_lib/Physical Signals/Sources/PS Constant  constant=apjbfyixny
  Redacted_9087 : PMIOPort  Side=Left
  Redacted_8009 : PMIOPort  Port=2  Side=Left
  Redacted_6326 : PMIOPort  Port=3  Side=Left
  Redacted_1150 : PMIOPort  Port=4  Side=Left
  Redacted_6426 : PMIOPort  Port=5  Side=Left
  Redacted_8072 : PMIOPort  Port=6  Side=Left
  Redacted_4470 : PMIOPort  Port=7  Side=Left
  Redacted_1909 : PMIOPort  Port=8  Side=Left
  Redacted_4712 : PMIOPort  Port=9  Side=Left
  Redacted_327 : PMIOPort  Port=10  Side=Left
  Redacted_3395 : PMIOPort  Port=11  Side=Left
  Redacted_6977 : PMIOPort  Port=12  Side=Left
  Redacted_4149 : PMIOPort  Port=13  Side=Left
  Redacted_8379 : PMIOPort  Port=14  Side=Left
  Redacted_6062 : PMIOPort  Port=15  Side=Left
  Redacted_8951 : PMIOPort  Port=16  Side=Left
  Redacted_7229 : PMIOPort  Port=17  Side=Left
  Redacted_3428 : PMIOPort  Port=18  Side=Left
  Redacted_7060 : PMIOPort  Port=19  Side=Left
  Redacted_6164 : PMIOPort  Port=20  Side=Left
  Redacted_8396 : PMIOPort  Port=21  Side=Left
  Redacted_9604 : PMIOPort  Port=22  Side=Left
  Redacted_4313 : PMIOPort  Port=23  Side=Left
  Redacted_8906 : PMIOPort  Port=24  Side=Left
  Redacted_3745 : PMIOPort  Port=25  Side=Left
  Redacted_1444 : PMIOPort  Port=26  Side=Left
  connections:
  Redacted_1444/RConn1 -- Redacted_9209/RConn2 -- Redacted_3564/RConn1
  Redacted_9763/LConn1 -- Redacted_5755/RConn1 -- Redacted_9763/LConn2
  Redacted_4470/RConn1 -- Redacted_3811/LConn1 -- Redacted_2625/LConn2
  Redacted_4355/RConn1 -- Redacted_7229/RConn1 -- Redacted_1169/RConn2
  Redacted_4759/LConn2 -- Redacted_3669/LConn2 -- Redacted_185/LConn2 -- Redacted_7011/LConn2 -- Redacted_7216/LConn2 -- Redacted_8664/LConn2 -- Redacted_7809/LConn2 -- Redacted_4255/LConn2 -- Redacted_8942/RConn1 -- Redacted_2852/LConn2
  Redacted_4352/LConn1 -- Redacted_6977/RConn1 -- Redacted_3288/LConn2
  Redacted_5647/RConn2 -- Redacted_8951/RConn1 -- Redacted_9315/RConn1
  Redacted_5755/LConn1 -- Redacted_4149/RConn1 -- Redacted_4697/LConn2
  Redacted_6609/RConn1 -- Redacted_7597/LConn2 -- Redacted_7597/LConn1
  Redacted_321/RConn1 -- Redacted_1243/LConn2 -- Redacted_1243/LConn1
  Redacted_5647/LConn1 -- Redacted_3395/RConn1 -- Redacted_9315/LConn2
  Redacted_8536/RConn1 -- Redacted_7508/LConn2 -- Redacted_7508/LConn1
  Redacted_1169/LConn1 -- Redacted_327/RConn1 -- Redacted_4355/LConn2
  Redacted_5756/RConn1 -- Redacted_2912/LConn2 -- Redacted_2912/LConn1
  Redacted_4352/RConn2 -- Redacted_6062/RConn1 -- Redacted_3288/RConn1
  Redacted_5647/RConn1 -- Redacted_3079/LConn2 -- Redacted_3079/LConn1
  Redacted_4352/RConn1 -- Redacted_2057/LConn2 -- Redacted_2057/LConn1
  Redacted_3716/RConn1 -- Redacted_7362/LConn2 -- Redacted_7362/LConn1
  Redacted_3811/RConn1 -- Redacted_5862/LConn2 -- Redacted_5862/LConn1
  Redacted_3174/RConn1 -- Redacted_5588/LConn2 -- Redacted_5588/LConn1
  Redacted_911/RConn1 -- Redacted_9991/LConn2 -- Redacted_9991/LConn1
  Redacted_5755/RConn2 -- Redacted_8379/RConn1 -- Redacted_4697/RConn1
  Redacted_1169/RConn1 -- Redacted_4828/LConn2 -- Redacted_4828/LConn1
  Redacted_3428/RConn1 -- Redacted_7273/RConn1 -- Redacted_5756/RConn2
  Redacted_4712/RConn1 -- Redacted_5756/LConn1 -- Redacted_7273/LConn2
  Redacted_8008/LConn1 -- Redacted_8008/LConn2 -- Redacted_9209/RConn1
  Redacted_9087/RConn1 -- Redacted_3564/LConn2 -- Redacted_9209/LConn1
  Redacted_8009/RConn1 -- Redacted_4565/LConn2 -- Redacted_3716/LConn1
  Redacted_6326/RConn1 -- Redacted_218/LConn2 -- Redacted_6609/LConn1
  Redacted_1150/RConn1 -- Redacted_911/LConn1 -- Redacted_6393/LConn2
  Redacted_6426/RConn1 -- Redacted_3174/LConn1 -- Redacted_2752/LConn2
  Redacted_8072/RConn1 -- Redacted_8536/LConn1 -- Redacted_8805/LConn2
  Redacted_1909/RConn1 -- Redacted_321/LConn1 -- Redacted_8383/LConn2
  Redacted_3745/RConn1 -- Redacted_4565/RConn1 -- Redacted_3716/RConn2
  Redacted_7060/RConn1 -- Redacted_321/RConn2 -- Redacted_8383/RConn1
  Redacted_6164/RConn1 -- Redacted_3811/RConn2 -- Redacted_2625/RConn1
  Redacted_8396/RConn1 -- Redacted_8536/RConn2 -- Redacted_8805/RConn1
  Redacted_9604/RConn1 -- Redacted_3174/RConn2 -- Redacted_2752/RConn1
  Redacted_4313/RConn1 -- Redacted_911/RConn2 -- Redacted_6393/RConn1
  Redacted_8906/RConn1 -- Redacted_6609/RConn2 -- Redacted_218/RConn1
  Redacted_5588/RConn1 -- Redacted_7011/LConn1
  Redacted_7597/RConn1 -- Redacted_8664/LConn1
  Redacted_4828/RConn1 -- Redacted_694/LConn1
  Redacted_9315/LConn1 -- Redacted_5457/RConn1
  Redacted_9991/RConn1 -- Redacted_7216/LConn1
  Redacted_2625/LConn1 -- Redacted_3669/RConn1
  Redacted_9395/RConn1 -- Redacted_5457/LConn2
  Redacted_2912/RConn1 -- Redacted_2852/LConn1
  Redacted_7273/LConn1 -- Redacted_2852/RConn1
  Redacted_1243/RConn1 -- Redacted_4759/LConn1
  Redacted_9763/RConn1 -- Redacted_4210/LConn1
  Redacted_8805/LConn1 -- Redacted_185/RConn1
  Redacted_7508/RConn1 -- Redacted_185/LConn1
  Redacted_3079/RConn1 -- Redacted_5457/LConn1
  Redacted_3039/RConn1 -- Redacted_4210/LConn2
  Redacted_4759/RConn1 -- Redacted_8383/LConn1
  Redacted_7809/RConn1 -- Redacted_4565/LConn1
  Redacted_3288/LConn1 -- Redacted_2786/RConn1
  Redacted_7362/RConn1 -- Redacted_7809/LConn1
  Redacted_5862/RConn1 -- Redacted_3669/LConn1
  Redacted_2057/RConn1 -- Redacted_2786/LConn1
  Redacted_218/LConn1 -- Redacted_8664/RConn1
  Redacted_2786/LConn2 -- Redacted_6432/RConn1
  Redacted_4355/LConn1 -- Redacted_694/RConn1
  Redacted_4210/RConn1 -- Redacted_4697/LConn1
  Redacted_7216/RConn1 -- Redacted_6393/LConn1
  Redacted_694/LConn2 -- Redacted_6051/RConn1
  Redacted_2752/LConn1 -- Redacted_7011/RConn1
  Redacted_8008/RConn1 -- Redacted_4255/LConn1
  Redacted_4255/RConn1 -- Redacted_3564/LConn1

== system Electrical_System_2018b_obfs/Redacted_4814/Redacted_3297/Redacted_8203 ==
  Redacted_{1695,3772,5153,6250} (4 alike) : nesl_utility/Solver Configuration  PhysicalDomain=network_engine_domain  SubClassName=solver  LeftPortType=input  RightPortType=generic  Tones=[]  Harmonics=[]  SimulateNoise=off  Profile=off  UseLocalSampling=off  EnableSwitchedLinearOptims=on  FrequencyDomain=off  UseCCode=off  RelTol=0.001  AbsTol=1e-06  MinStep=1e-09  ToWorkspace=off  RevertToSquareIcSolve=off  NumHomotopyIterations=100  PhasorMode=off  PhasorModeNumHarmonics=1  DoDC=off  ResidualTolerance=1e-09  UseLocalSolver=off  LocalSolverChoice=NE_BACKWARD_EULER_ADVANCER  LocalSolverSampleTime=0.001  DoFixedCost=off  MaxNonlinIter=3  MaxModeIter=2  LinearAlgebra=auto  EquationFormulation=NE_TIME_EF  DelaysMemoryBudget=1024  AutomaticFiltering=on  FilteringTimeConstant=0.001  PartitionStorageMethod=AS_NEEDED  PartitionMemoryBudget=1024  PartitionMethod=ROBUST
  Redacted_2385 : fl_lib/Physical Signals/Sources/PS Constant  constant=swmfzbxvsi
  Redacted_2431 : fl_lib/Mechanical/Rotational Elements/Mechanical Rotational Reference
  Redacted_2778 : fl_lib/Physical Signals/Sources/PS Constant  constant=mzfdazupnh
  Redacted_2918 : fl_lib/Mechanical/Rotational Elements/Mechanical Rotational Reference
  Redacted_2927 : fl_lib/Physical Signals/Sources/PS Constant  constant=qrqipbnjkc
  Redacted_2937 : fl_lib/Physical Signals/Sources/PS Constant  constant=bklwjikrlr
  Redacted_4172 : fl_lib/Gas/Elements/Controlled Reservoir (G)  area_A=xpmpvwsckg m^2
      settings: SourceProductName=Simscape  SourceProductBaseCode=SS  InternalSimscapePortConfiguration="{\"Bottom\":[],\"Left\":[{\"id\":\"A\",\"label\":\"A\",\"type\":\"foundation.gas.gas\"}],\"Right\":[{\"id\":\"T_in\",\"label\":\"T\",\"type\":\"input\"},{\"id\":\"p_in\",\"label\":\"P\",\"type\":\"input\"}],\"Top\":[]}"
  Redacted_4198 : fl_lib/Physical Signals/Sources/PS Constant  constant=tigdeznnel
  Redacted_4563 : fl_lib/Gas/Elements/Controlled Reservoir (G)  area_A=dqdrcthbbg m^2
      settings: SourceProductName=Simscape  SourceProductBaseCode=SS  InternalSimscapePortConfiguration="{\"Bottom\":[],\"Left\":[{\"id\":\"A\",\"label\":\"A\",\"type\":\"foundation.gas.gas\"}],\"Right\":[{\"id\":\"T_in\",\"label\":\"T\",\"type\":\"input\"},{\"id\":\"p_in\",\"label\":\"P\",\"type\":\"input\"}],\"Top\":[]}"
  Redacted_5008 : fl_lib/Physical Signals/Sources/PS Constant  constant=aabgypnlfs
  Redacted_7202 : fl_lib/Mechanical/Mechanical Sources/Ideal Angular Velocity Source
  Redacted_9927 : fl_lib/Mechanical/Mechanical Sources/Ideal Angular Velocity Source
  Redacted_6460 : PMIOPort  Side=Right
  Redacted_4230 : PMIOPort  Port=2  Side=Right
  Redacted_9119 : PMIOPort  Port=3  Side=Right
  Redacted_901 : PMIOPort  Port=4  Side=Right
  connections:
  Redacted_9927/LConn1 -- Redacted_1695/RConn1 -- Redacted_9119/RConn1
  Redacted_6460/RConn1 -- Redacted_3772/RConn1 -- Redacted_7202/LConn1
  Redacted_4172/LConn1 -- Redacted_6250/RConn1 -- Redacted_4230/RConn1
  Redacted_901/RConn1 -- Redacted_5153/RConn1 -- Redacted_4563/LConn1
  Redacted_2918/LConn1 -- Redacted_9927/RConn2
  Redacted_2927/RConn1 -- Redacted_9927/RConn1
  Redacted_7202/RConn1 -- Redacted_2385/RConn1
  Redacted_2431/LConn1 -- Redacted_7202/RConn2
  Redacted_4172/RConn2 -- Redacted_2778/RConn1
  Redacted_4172/RConn1 -- Redacted_5008/RConn1
  Redacted_4563/RConn2 -- Redacted_2937/RConn1
  Redacted_4198/RConn1 -- Redacted_4563/RConn1
